simulink library "breakers_1ph_3ph"  (R2013a)
settings: Solver=ode45  StartTime=0.0  StopTime=10.0  RelTol=1e-3
undefined symbols (not defined in the file): DiscIntNeverNeededParam, IOC, sim_Freq_Hz, TOC, TOC_T, Ts
libraries: simulink x8, powerlib_extras x7, breakers_1ph_3ph x4, simulink_extras x4, powerlib x4, dspsigops x3
settings Model: Creator=re25624  LastModifiedBy=ed12083

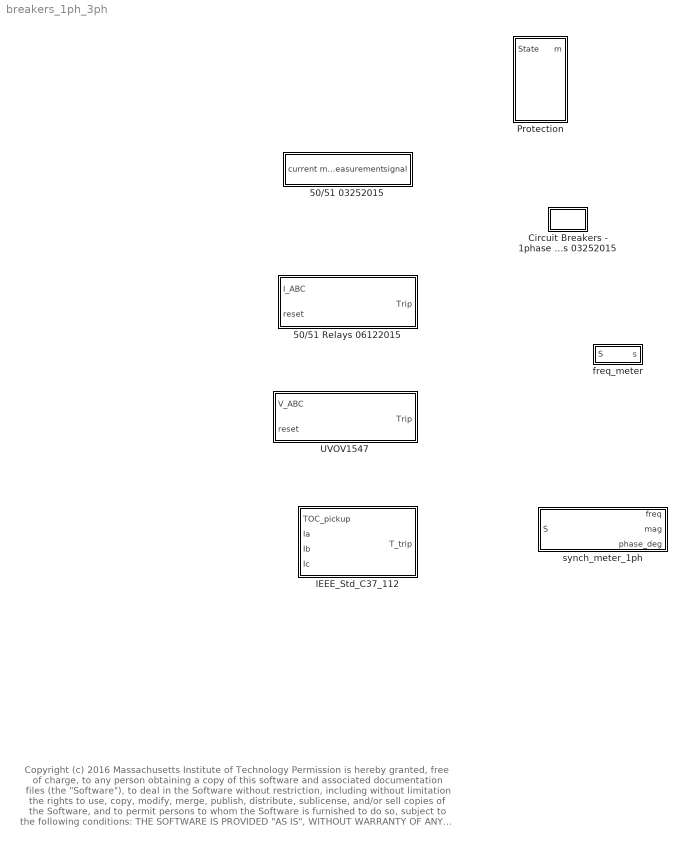
== system breakers_1ph_3ph ==
  note: Copyright (c) 2016 Massachusetts Institute of Technology
      | Permission is hereby granted, free of charge, to any person obtaining a copy of this software and associated documentation files (the "Software"), to deal
      | in the Software without restriction, including without limitation the rights to use, copy, modify, merge, publish, distribute, sublicense, and/or sell copies of the
      | Software, and to permit persons to whom the Software is furnished to do so, subject to the following conditions:
      |
      | THE SOFTWARE IS PROVIDED "AS IS", WITHOUT WARRANTY OF ANY KIND, EXPRESS OR IMPLIED, INCLUDING BUT NOT LIMITED TO THE
      | WARRANTIES OF MERCHANTABILITY, FITNESS FOR A PARTICULAR PURPOSE AND NONINFRINGEMENT. IN NO EVENT SHALL THE AUTHORS
      | OR COPYRIGHT HOLDERS BE LIABLE FOR ANY CLAIM, DAMAGES OR OTHER LIABILITY, WHETHER IN AN ACTION OF CONTRACT, TORT OR
      | OTHERWISE, ARISING FROM, OUT OF OR IN CONNECTION WITH THE SOFTWARE OR THE USE OR OTHER DEALINGS IN THE SOFTWARE
  50/51 03252015 : Subsystem  mask{IOC=IOC, TOC=TOC, TOC_T=TOC_T, Ts=Ts, sim_Freq_Hz=sim_Freq_Hz}
      mask prompts: IOC "IOC [A]"; TOC "TOC [A]"; TOC_T "TOC Delay [Sec]"; Ts "Sampling Time"; sim_Freq_Hz "Frequency [Hz]"
      mask help: This is a very simple model of instantaneous overcurrent and the inverse time overcurrent relays (50/51). It is not suitable for instantaneous earth current relaying. The model neglects the influence CTs since only the logics of the relay are required or the current effort. The input parameters to the model are: measured line current, sampling time (Ts) and simulation frequency (sim_Freq_Hz)
  50/51 Relays 06122015 : Subsystem  mask(50/51 Relays){TOC=150, IOC=900, Ts=Ts}
      mask prompts: TOC "TOC [A]"; IOC "IOC [A]"; Ts "Sampling Time [Secs]"
      mask help:
      | This is a model of instantaneous overcurrent and the inverse time overcurrent relays (50/51).
      | It is not suitable for instantaneous earth current relaying.
      | The model neglects the influence CTs since only the logics of the relay are required or the current effort.
      | The input parameters to the model are: measured line current, and sampling time (Ts)
  Circuit Breakers - 1phase with 50/51 relays 03252015 : Subsystem  mask{IOC=3000, TOC=600, TOC_T=0.1, MECH_T=0.05, open_command=1E15, close_command=1E15, sim_Freq_Hz=60, Ts=50e-6}
      mask prompts: IOC "IOC setting [A]"; TOC "TOC setting [A]"; TOC_T "TOC time dealy [Sec]"; MECH_T "Mechanical time delay [Sec]"; open_command "Manual open time [Sec]"; close_command "Manual close time [Sec]"; sim_Freq_Hz "Frequency [Hz]"; Ts "Sampling Time"
  IEEE_Std_C37_112 : Subsystem
  Protection : Subsystem  mask(Protection and Metering){IOC=7200, TOC=1920, Ts=50E-6}
      mask prompts: IOC "IOC setting [A]"; TOC "TOC setting [A]"; Ts "Sampling Time"
      mask help:
      | This block simulates the behavior of selected relay functions as well as metering equipment.
      | The block is intended to communicate with a microgrid controller providing it measurements, and switching controls.
      |
      | Supported relay functions (as of 06-15-2015):
      | 50/51: instantaneous and time-inverse overcurrent protection (moderate curve)
      mask Help:
      | This block simulates the behavior of selected relay functions as well as metering equipment (60 Hz - only).
      | The block is intended to communicate with a microgrid controller providing it measurements, and switching controls.
      | 
      | Supported relay functions (as of 06-15-2015):
      | 50/51: instantaneous and time-inverse overcurrent protection (moderate curve)
      | 
      | The input parameters are:
      | 0) Ts:  Sampling time [Seconds]
      | 1) State: 0 for relay logic mode, 1 to close the controlled breaker/switch,
      | and 2 to open the controlled breaker/switch
      | 2) TOC: Time-inverse overcurrent setting [Amperes]
      | 3) IOC: Instantaneous overcurrent setting [Amperes]
      | 
      | Metered parameters are:
      | 0) Status (0-closed, 1-open)
      | 1) Instantaneous voltage (abc)
      | 2) Instantaneous current (abc)
  UVOV1547 : Subsystem  mask(IEEE Std. 1457 UVOV Protection){VRMSLL=13800, Ts=Ts}
      mask prompts: VRMSLL "Nominal Voltage [VRMSLL]"; Ts "Sampling Time, [Secs]"
      mask help:
      | This is a model of the IEEE Std. 1457 undervoltage and overvoltage protection check.
      | The model neglects the influence PTs since only the logics of the relay are required or the current effort.
      | The input parameters to the model are: measured voltage RMSLL, and sampling time (Ts)
  freq_meter : Subsystem  mask(Frequency Meter){Ts=Ts}
      mask prompts: Ts "Time Step, Ts [Sec]"
      mask help:
      | This block measures the frequency of and input signal (voltage, current, etc) at the rising edge of zero-crossing. There more advanced and efficient methods to meter frequency (i.e. DFT). However, most of the relays in the power system operate on the principle of zero crossing detection.
      |
      | ** The error in measurement is relative to the specified time step. It is recommended Ts <= 80E-6 s.
  synch_meter_1ph : Subsystem  mask(Synchronizer meter){Ts=Ts}
      mask prompts: Ts "Time Step, Ts [sec]"
      mask help:
      | This block measures frequency, magnitude and phase of an input signal. Requires one cycle to initialize.
      | **** The error in measurement of the internal components is relative to the specified time step. It is recommended Ts <= 80E-6 s.

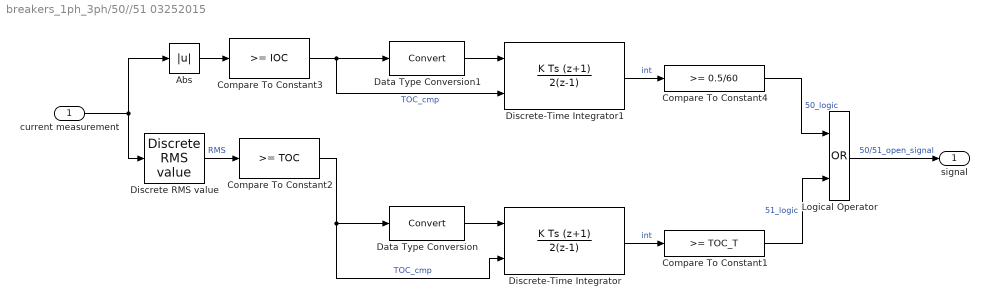
== system breakers_1ph_3ph/50//51 03252015 ==
  current measurement : Inport
  Abs : Abs
  Compare To Constant1 : simulink/Logic and Bit Operations/Compare To Constant  relop=>=  const=TOC_T  OutDataTypeStr=boolean
  Compare To Constant2 : simulink/Logic and Bit Operations/Compare To Constant  relop=>=  const=TOC  OutDataTypeStr=boolean
  Compare To Constant3 : simulink/Logic and Bit Operations/Compare To Constant  relop=>=  const=IOC  OutDataTypeStr=boolean
  Compare To Constant4 : simulink/Logic and Bit Operations/Compare To Constant  relop=>=  const=0.5/60  OutDataTypeStr=boolean
  Data Type Conversion : DataTypeConversion
  Data Type Conversion1 : DataTypeConversion
  Discrete RMS value : powerlib_extras/Discrete Measurements/Discrete  RMS value  Freq=60  Mag_Init=0  Ts=Ts
  Discrete-Time Integrator : DiscreteIntegrator  IntegratorMethod=Integration: Trapezoidal  ExternalReset=falling  InitialConditionMode=State only (most efficient)  SampleTime=-1  ICPrevOutput=DiscIntNeverNeededParam  ICPrevScaledInput=DiscIntNeverNeededParam
  Discrete-Time Integrator1 : DiscreteIntegrator  IntegratorMethod=Integration: Trapezoidal  ExternalReset=falling  InitialConditionMode=State only (most efficient)  SampleTime=-1  ICPrevOutput=DiscIntNeverNeededParam  ICPrevScaledInput=DiscIntNeverNeededParam
  Logical Operator : Logic  Operator=OR  AllPortsSameDT=off  OutDataTypeStr=boolean
  signal : Outport
  wires:
  Logical Operator/1 -> signal/1  "50/51_open_signal"
  Compare To Constant1/1 -> Logical Operator/2  "51_logic"
  Abs/1 -> Compare To Constant3/1
  Discrete RMS value/1 -> Compare To Constant2/1  "RMS"
  Data Type Conversion/1 -> Discrete-Time Integrator/1
  Discrete-Time Integrator/1 -> Compare To Constant1/1  "int"
  current measurement/1 -> Abs/1, Discrete RMS value/1
  Compare To Constant2/1 -> Discrete-Time Integrator/2, Data Type Conversion/1  "TOC_cmp"
  Data Type Conversion1/1 -> Discrete-Time Integrator1/1
  Discrete-Time Integrator1/1 -> Compare To Constant4/1  "int"
  Compare To Constant3/1 -> Discrete-Time Integrator1/2, Data Type Conversion1/1  "TOC_cmp"
  Compare To Constant4/1 -> Logical Operator/1  "50_logic"

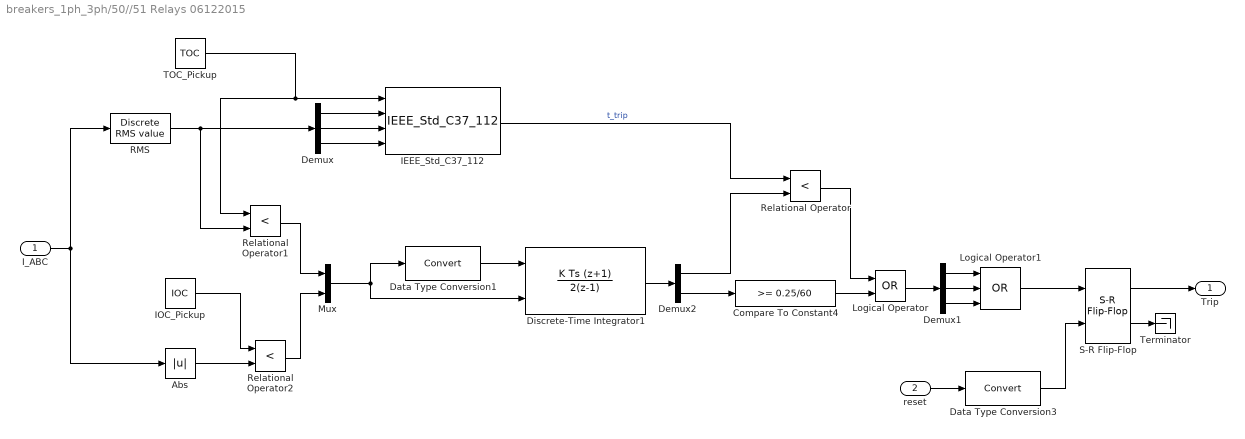
== system breakers_1ph_3ph/50//51 Relays 06122015 ==
  I_ABC : Inport
  reset : Inport  Port=2
  Abs : Abs
  Compare To Constant4 : simulink/Logic and Bit Operations/Compare To Constant  relop=>=  const=0.25/60  OutDataTypeStr=boolean
  Data Type Conversion1 : DataTypeConversion
  Data Type Conversion3 : DataTypeConversion
  Demux : Demux  Outputs=3
  Demux1 : Demux  Outputs=3
  Demux2 : Demux  Outputs=2
  Discrete-Time Integrator1 : DiscreteIntegrator  IntegratorMethod=Integration: Trapezoidal  ExternalReset=falling  InitialConditionMode=State only (most efficient)  SampleTime=-1  ICPrevOutput=DiscIntNeverNeededParam  ICPrevScaledInput=DiscIntNeverNeededParam
  IEEE_Std_C37_112 : breakers_1ph_3ph/IEEE_Std_C37_112
  IOC_Pickup : Constant  Value=IOC
  Logical Operator : Logic  Operator=OR  AllPortsSameDT=off  OutDataTypeStr=boolean
  Logical Operator1 : Logic  Operator=OR  Inputs=3  AllPortsSameDT=off  OutDataTypeStr=boolean
  Mux : Mux  Inputs=2
  RMS : powerlib_extras/Discrete Measurements/Discrete  RMS value  Freq=60  Mag_Init=0  Ts=Ts
  Relational Operator : RelationalOperator  Operator=<  OutDataTypeStr=boolean
  Relational Operator1 : RelationalOperator  Operator=<  OutDataTypeStr=boolean
  Relational Operator2 : RelationalOperator  Operator=<  OutDataTypeStr=boolean
  S-R Flip-Flop : simulink_extras/Flip Flops/S-R Flip-Flop  initial_condition=0
  TOC_Pickup : Constant  Value=TOC
  Terminator : Terminator
  Trip : Outport
  wires:
  Demux2/2 -> Compare To Constant4/1
  Demux2/1 -> Relational Operator/2
  Discrete-Time Integrator1/1 -> Demux2/1
  Mux/1 -> Discrete-Time Integrator1/2, Data Type Conversion1/1
  Relational Operator2/1 -> Mux/2
  Relational Operator1/1 -> Mux/1
  Data Type Conversion3/1 -> S-R Flip-Flop/2
  reset/1 -> Data Type Conversion3/1
  Logical Operator1/1 -> S-R Flip-Flop/1
  Demux1/3 -> Logical Operator1/3
  Demux1/2 -> Logical Operator1/2
  Demux1/1 -> Logical Operator1/1
  Logical Operator/1 -> Demux1/1
  S-R Flip-Flop/2 -> Terminator/1
  S-R Flip-Flop/1 -> Trip/1
  I_ABC/1 -> RMS/1, Abs/1
  TOC_Pickup/1 -> Relational Operator1/1, IEEE_Std_C37_112/1
  Demux/3 -> IEEE_Std_C37_112/4
  Demux/2 -> IEEE_Std_C37_112/3
  Demux/1 -> IEEE_Std_C37_112/2
  RMS/1 -> Relational Operator1/2, Demux/1
  IOC_Pickup/1 -> Relational Operator2/1
  Relational Operator/1 -> Logical Operator/1
  Compare To Constant4/1 -> Logical Operator/2
  Abs/1 -> Relational Operator2/2
  IEEE_Std_C37_112/1 -> Relational Operator/1  "t_trip"
  Data Type Conversion1/1 -> Discrete-Time Integrator1/1

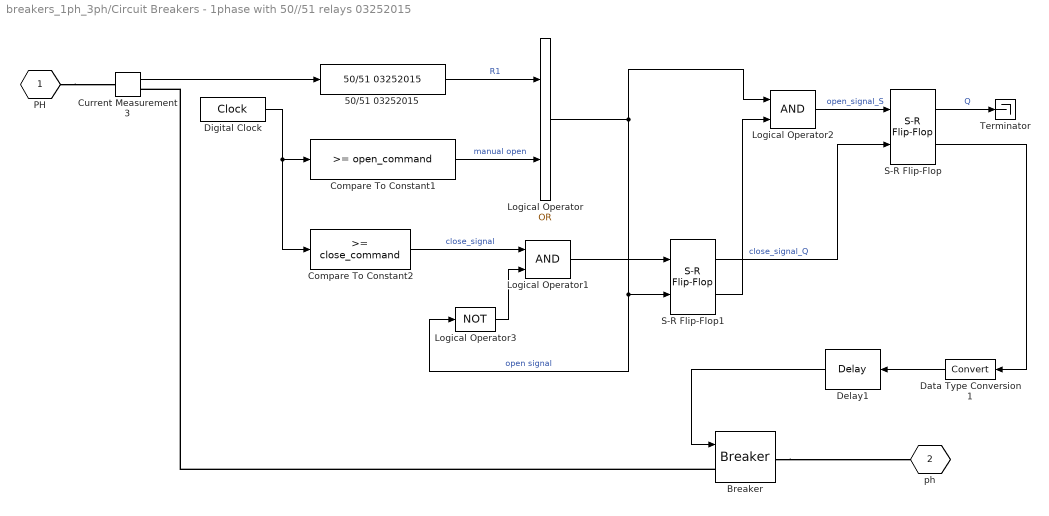
== system breakers_1ph_3ph/Circuit Breakers - 1phase with 50//51 relays 03252015 ==
  50/51 03252015 : breakers_1ph_3ph/50//51 03252015  IOC=IOC  TOC=TOC  TOC_T=TOC_T  Ts=Ts  sim_Freq_Hz=sim_Freq_Hz
  Breaker : powerlib/Elements/Breaker  BreakerResistance=1e-3  InitialState=1  SnubberResistance=1e6  SnubberCapacitance=inf  SwitchingTimes="[1/60  5/60]"  External=on  Measurements=None  MoreParameters=on  NoBreakLoop=off
  Compare To Constant1 : simulink/Logic and Bit Operations/Compare To Constant  relop=>=  const=open_command  OutDataTypeStr=boolean
  Compare To Constant2 : simulink/Logic and Bit Operations/Compare To Constant  relop=>=  const=close_command  OutDataTypeStr=boolean
  Current Measurement3 : powerlib/Measurements/Current Measurement  PhasorSimulation=off  OutputType=Complex  PSBequivalent=0
  Data Type Conversion1 : DataTypeConversion
  Delay1 : dspsigops/Delay  dly_unit=Samples  delay=lower(MECH_T/Ts)  ic_detail=off  dif_ic_for_ch=off  dif_ic_for_dly=off  ic=1  reset_popup=None
  Digital Clock : DigitalClock  SampleTime=Ts
  Logical Operator : Logic  Operator=OR  AllPortsSameDT=off  OutDataTypeStr=boolean
  Logical Operator1 : Logic  AllPortsSameDT=off  OutDataTypeStr=boolean
  Logical Operator2 : Logic  AllPortsSameDT=off  OutDataTypeStr=boolean
  Logical Operator3 : Logic  Operator=NOT  AllPortsSameDT=off  OutDataTypeStr=boolean
  S-R Flip-Flop : simulink_extras/Flip Flops/S-R Flip-Flop  initial_condition=0
  S-R Flip-Flop1 : simulink_extras/Flip Flops/S-R Flip-Flop  initial_condition=0
  Terminator : Terminator
  PH : PMIOPort  Tag=PMCPort  Port=1  Side=Left
  ph : PMIOPort  Tag=PMCPort  Port=2  Side=Right
  wires:
  Delay1/1 -> Breaker/1
  Logical Operator1/1 -> S-R Flip-Flop1/1
  Compare To Constant2/1 -> Logical Operator1/1  "close_signal"
  Logical Operator/1 -> S-R Flip-Flop1/2, Logical Operator3/1, Logical Operator2/1  "open signal"
  S-R Flip-Flop1/1 -> S-R Flip-Flop/2  "close_signal_Q"
  S-R Flip-Flop/2 -> Data Type Conversion1/1
  S-R Flip-Flop1/2 -> Logical Operator2/2
  Compare To Constant1/1 -> Logical Operator/2  "manual open"
  Logical Operator3/1 -> Logical Operator1/2
  Digital Clock/1 -> Compare To Constant1/1, Compare To Constant2/1
  50/51 03252015/1 -> Logical Operator/1  "R1"
  S-R Flip-Flop/1 -> Terminator/1  "Q"
  Current Measurement3/1 -> 50/51 03252015/1
  Logical Operator2/1 -> S-R Flip-Flop/1  "open_signal_S"
  Data Type Conversion1/1 -> Delay1/1
  connections:
  Breaker/RConn1 -- ph/RConn1
  PH/RConn1 -- Current Measurement3/LConn1
  Breaker/LConn1 -- Current Measurement3/RConn1

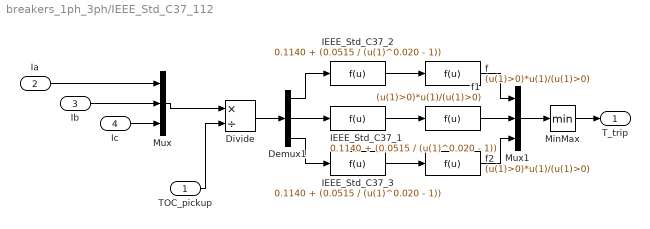
== system breakers_1ph_3ph/IEEE_Std_C37_112 ==
  TOC_pickup : Inport
  Ia : Inport  Port=2
  Ib : Inport  Port=3
  Ic : Inport  Port=4
  Demux1 : Demux  Outputs=3
  Divide : Product  Inputs=*/
  IEEE_Std_C37_1 : Fcn  Expr=0.1140 + (0.0515 / (u(1)^0.020 - 1))
  IEEE_Std_C37_2 : Fcn  Expr=0.1140 + (0.0515 / (u(1)^0.020 - 1))
  IEEE_Std_C37_3 : Fcn  Expr=0.1140 + (0.0515 / (u(1)^0.020 - 1))
  MinMax : MinMax
  Mux : Mux  Inputs=3
  Mux1 : Mux  Inputs=3
  f : Fcn  Expr=(u(1)>0)*u(1)/(u(1)>0)
  f1 : Fcn  Expr=(u(1)>0)*u(1)/(u(1)>0)
  f2 : Fcn  Expr=(u(1)>0)*u(1)/(u(1)>0)
  T_trip : Outport
  wires:
  Ic/1 -> Mux/3
  TOC_pickup/1 -> Divide/2
  MinMax/1 -> T_trip/1
  Ib/1 -> Mux/2
  Ia/1 -> Mux/1
  f2/1 -> Mux1/3
  f1/1 -> Mux1/2
  f/1 -> Mux1/1
  Mux/1 -> Divide/1
  Mux1/1 -> MinMax/1
  IEEE_Std_C37_3/1 -> f2/1
  IEEE_Std_C37_1/1 -> f1/1
  IEEE_Std_C37_2/1 -> f/1
  Divide/1 -> Demux1/1
  Demux1/3 -> IEEE_Std_C37_3/1
  Demux1/2 -> IEEE_Std_C37_1/1
  Demux1/1 -> IEEE_Std_C37_2/1

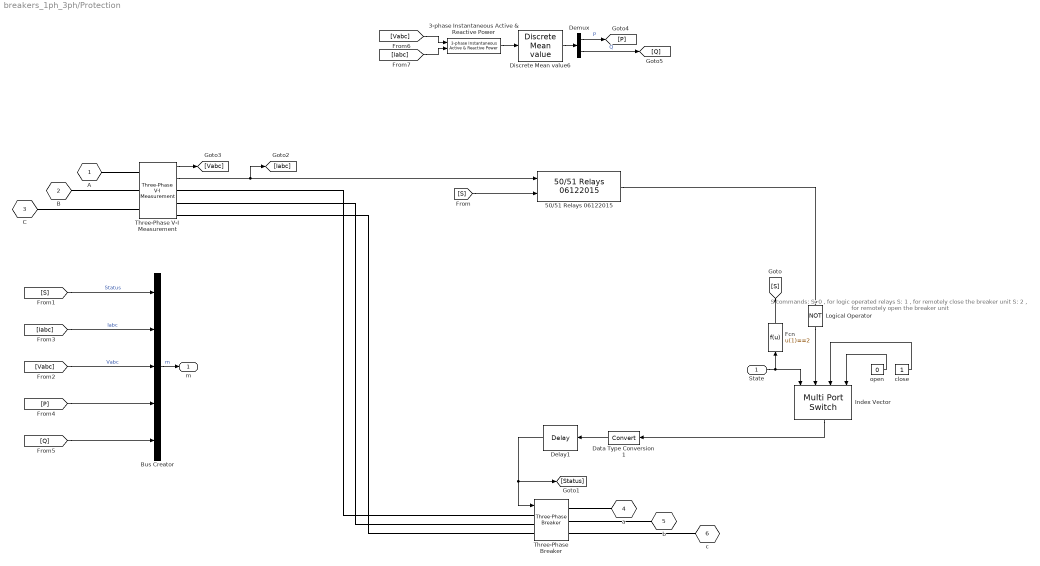
== system breakers_1ph_3ph/Protection ==
  note: S commands:
      | S: 0 , for logic operated relays
      | S: 1 ,  for remotely close the breaker unit
      | S: 2 , for remotely open the breaker unit
  State : Inport
  3-phase Instantaneous Active & Reactive Power : powerlib_extras/Measurements/3-phase  Instantaneous  Active & Reactive Power
  50/51 Relays 06122015 : breakers_1ph_3ph/50//51 Relays 06122015  TOC=TOC  IOC=IOC  Ts=Ts
  Bus Creator : BusCreator  Inputs=5
  Data Type Conversion1 : DataTypeConversion
  Delay1 : dspsigops/Delay  dly_unit=Samples  delay=lower((3/60)/Ts)  ic_detail=off  dif_ic_for_ch=off  dif_ic_for_dly=off  ic=1  reset_popup=None
  Demux : Demux  Outputs=2
  Discrete Mean value6 : powerlib_extras/Discrete Measurements/Discrete  Mean value  Freq=60  Vinit=0  Ts=Ts
  Fcn : Fcn  Expr=u(1)==2
  Index Vector : MultiPortSwitch  DataPortOrder=Zero-based contiguous  DataPortIndices={2,1,0}  zeroidx=on
  Logical Operator : Logic  Operator=NOT  AllPortsSameDT=off  OutDataTypeStr=boolean
  Three-Phase V-I Measurement : powerlib/Measurements/Three-Phase V-I Measurement  VoltageMeasurement=phase-to-ground  SetLabelV=off  LabelV=Vabc  Vpu=off  VpuLL=off  CurrentMeasurement=yes  SetLabelI=off  LabelI=Iabc  Ipu=off  Pbase=100e6  Vbase=500e3  OutputType=Complex  PhasorSimulation=off  PSBequivalent=0
  Three-Phase Breaker : powerlib/Elements/Three-Phase Breaker  InitialState=closed  SwitchA=on  SwitchB=on  SwitchC=on  SwitchTimes="[1/60  5/60]"  External=on  BreakerResistance=1e-3  SnubberResistance=1e6  SnubberCapacitance=1e-12  Measurements=None
  close : Constant
  open : Constant  Value=0
  A : PMIOPort  Tag=PMCPort  Port=1  Side=Left
  B : PMIOPort  Tag=PMCPort  Port=2  Side=Left
  C : PMIOPort  Tag=PMCPort  Port=3  Side=Left
  a : PMIOPort  Tag=PMCPort  Port=4  Side=Right
  b : PMIOPort  Tag=PMCPort  Port=5  Side=Right
  c : PMIOPort  Tag=PMCPort  Port=6  Side=Right
  m : Outport
  wires:
  Data Type Conversion1/1 -> Delay1/1
  Index Vector/1 -> Data Type Conversion1/1
  State/1 -> Index Vector/1, Fcn/1
  close/1 -> Index Vector/3
  open/1 -> Index Vector/4
  Three-Phase V-I Measurement/2 -> 50/51 Relays 06122015/1, [Iabc]
  Three-Phase V-I Measurement/1 -> [Vabc]
  Delay1/1 -> Three-Phase Breaker/1, [Status]
  [S] -> 50/51 Relays 06122015/2
  [S] -> Bus Creator/1  "Status"
  Bus Creator/1 -> m/1  "m"
  Fcn/1 -> [S]
  Logical Operator/1 -> Index Vector/2
  50/51 Relays 06122015/1 -> Logical Operator/1
  Discrete Mean value6/1 -> Demux/1
  3-phase Instantaneous Active & Reactive Power/1 -> Discrete Mean value6/1
  Demux/2 -> [Q]  "Q"
  Demux/1 -> [P]  "P"
  [Iabc] -> Bus Creator/2  "Iabc"
  [Vabc] -> Bus Creator/3  "Vabc"
  [Iabc] -> 3-phase Instantaneous Active & Reactive Power/2
  [Vabc] -> 3-phase Instantaneous Active & Reactive Power/1
  [P] -> Bus Creator/4
  [Q] -> Bus Creator/5
  connections:
  B/RConn1 -- Three-Phase V-I Measurement/LConn2
  C/RConn1 -- Three-Phase V-I Measurement/LConn3
  a/RConn1 -- Three-Phase Breaker/RConn1
  Three-Phase V-I Measurement/LConn1 -- A/RConn1
  Three-Phase Breaker/RConn3 -- c/RConn1
  Three-Phase Breaker/RConn2 -- b/RConn1
  Three-Phase Breaker/LConn3 -- Three-Phase V-I Measurement/RConn3
  Three-Phase Breaker/LConn2 -- Three-Phase V-I Measurement/RConn2
  Three-Phase Breaker/LConn1 -- Three-Phase V-I Measurement/RConn1

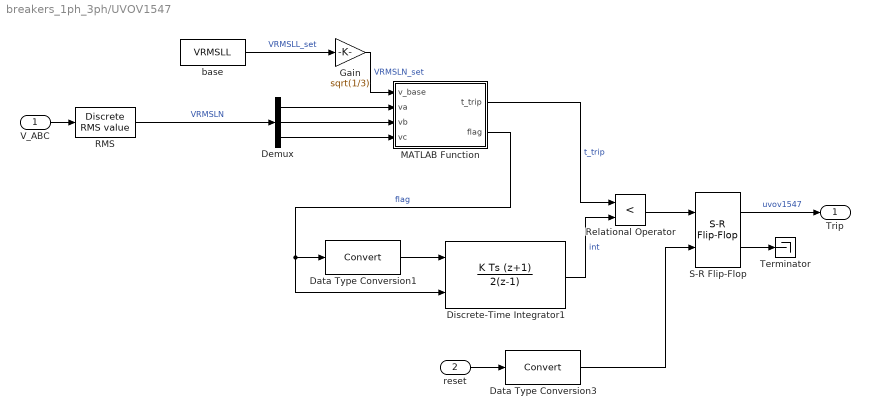
== system breakers_1ph_3ph/UVOV1547 ==
  V_ABC : Inport
  reset : Inport  Port=2
  Data Type Conversion1 : DataTypeConversion
  Data Type Conversion3 : DataTypeConversion
  Demux : Demux  Outputs=3
  Discrete-Time Integrator1 : DiscreteIntegrator  IntegratorMethod=Integration: Trapezoidal  ExternalReset=falling  InitialConditionMode=State only (most efficient)  SampleTime=-1  ICPrevOutput=DiscIntNeverNeededParam  ICPrevScaledInput=DiscIntNeverNeededParam
  Gain : Gain  Gain=sqrt(1/3)
  MATLAB Function : MATLAB Function  TreatAsAtomicUnit=on
  RMS : powerlib_extras/Discrete Measurements/Discrete  RMS value  Freq=60  Mag_Init=VRMSLL*sqrt(1/3)  Ts=Ts
  Relational Operator : RelationalOperator  Operator=<  OutDataTypeStr=boolean
  S-R Flip-Flop : simulink_extras/Flip Flops/S-R Flip-Flop  initial_condition=0
  Terminator : Terminator
  base : Constant  Value=VRMSLL
  Trip : Outport
  wires:
  V_ABC/1 -> RMS/1
  Relational Operator/1 -> S-R Flip-Flop/1
  MATLAB Function/2(flag) -> Discrete-Time Integrator1/2, Data Type Conversion1/1  "flag"
  Gain/1 -> MATLAB Function/1(v_base)  "VRMSLN_set"
  Discrete-Time Integrator1/1 -> Relational Operator/2  "int"
  Data Type Conversion3/1 -> S-R Flip-Flop/2
  reset/1 -> Data Type Conversion3/1
  S-R Flip-Flop/2 -> Terminator/1
  S-R Flip-Flop/1 -> Trip/1  "uvov1547"
  base/1 -> Gain/1  "VRMSLL_set"
  Demux/3 -> MATLAB Function/4(vc)
  Demux/2 -> MATLAB Function/3(vb)
  Demux/1 -> MATLAB Function/2(va)
  RMS/1 -> Demux/1  "VRMSLN"
  MATLAB Function/1(t_trip) -> Relational Operator/1  "t_trip"
  Data Type Conversion1/1 -> Discrete-Time Integrator1/1

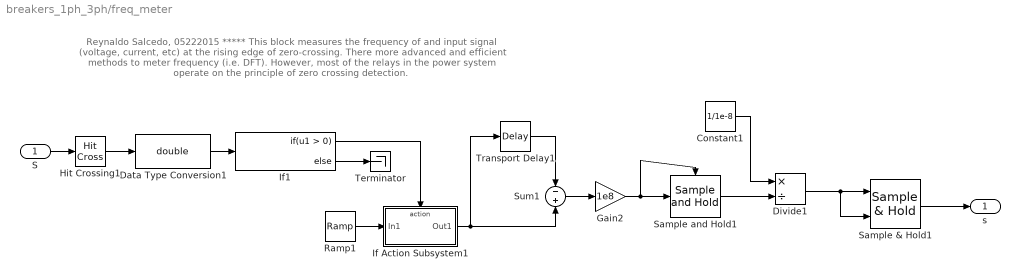
== system breakers_1ph_3ph/freq_meter ==
  note: Reynaldo Salcedo, 05222015
      | ***** This block measures the frequency of and input signal (voltage, current, etc) at the rising edge of zero-crossing.
      | There more advanced and efficient methods to meter frequency (i.e. DFT).
      | However, most of the relays in the power system operate on the principle of zero crossing detection.
  S : Inport
  Constant1 : Constant  Value=1/1e-8
  Data Type Conversion1 : DataTypeConversion  OutDataTypeStr=double
  Divide1 : Product  Inputs=*/
  Gain2 : Gain  Gain=1e8
  Hit Crossing1 : HitCross  HitCrossingDirection=rising
  If Action Subsystem1 : Subsystem  TreatAsAtomicUnit=on
  If1 : If
  Ramp1 : simulink/Sources/Ramp  slope=1  start=0  X0=60
  Sample and Hold1 : dspsigops/Sample and Hold  trig=Rising edge  initCond=0  latchinput=off
  Sample & Hold1 : powerlib_extras/Control  Blocks/Sample & Hold  ic=0
  Sum1 : Sum  Inputs=-+
  Terminator : Terminator
  Transport Delay1 : TransportDelay  DelayTime=Ts
  s : Outport
  wires:
  Sample and Hold1/1 -> Divide1/2
  Divide1/1 -> Sample & Hold1/2, Sample & Hold1/1
  If1/2 -> Terminator/1
  If1/1 -> If Action Subsystem1/Action
  Sample & Hold1/1 -> s/1
  Constant1/1 -> Divide1/1
  Gain2/1 -> Sample and Hold1/Trigger, Sample and Hold1/1
  Sum1/1 -> Gain2/1
  Transport Delay1/1 -> Sum1/1
  If Action Subsystem1/1(Out1) -> Sum1/2, Transport Delay1/1
  Ramp1/1 -> If Action Subsystem1/1(In1)
  Hit Crossing1/1 -> Data Type Conversion1/1
  Data Type Conversion1/1 -> If1/1
  S/1 -> Hit Crossing1/1

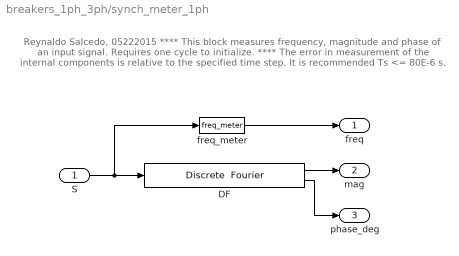
== system breakers_1ph_3ph/synch_meter_1ph ==
  note: Reynaldo Salcedo, 05222015
      | **** This block measures frequency, magnitude and phase of an input signal.
      | Requires one cycle to initialize.
      | **** The error in measurement of the internal components is relative to the specified time step. It is recommended Ts <= 80E-6 s.
  S : Inport
  DF : powerlib_extras/Discrete Measurements/Discrete  Fourier  Freq=60  n=1  Par_Init=[0 0]  Ts=Ts
  freq_meter : breakers_1ph_3ph/freq_meter  Ts=Ts
  freq : Outport
  mag : Outport  Port=2
  phase_deg : Outport  Port=3
  wires:
  S/1 -> DF/1, freq_meter/1
  freq_meter/1 -> freq/1
  DF/2 -> phase_deg/1
  DF/1 -> mag/1

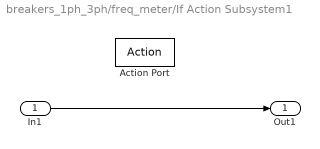
== system breakers_1ph_3ph/freq_meter/If Action Subsystem1 ==
  In1 : Inport
  Action Port : ActionPort
  Out1 : Outport
  wires:
  In1/1 -> Out1/1

== matlab function breakers_1ph_3ph/UVOV1547/MATLAB Function ==
  data: v_base input; va input; t_trip output; vb input; vc input; flag output
function [t_trip, flag] = uvov1547(v_base,va,vb,vc)
%#codegen

v_pu = [va, vb, vc] ./ v_base;
mech_delay = 3/60;
t = 1E6;
flag = 0;

% IEEE Std 1547a-2014 (Amendment to IEEE Std 1547-2003)
% Table 1-Interconnection system default response to abnormal voltages

if max(v_pu < 0.45)
    t=0.16;
    flag=1;
elseif max(v_pu >= 0.45) && max(v_pu < 0.60)
    t=1;
    flag=1;
elseif max(v_pu >= 0.60) && max(v_pu < 0.88)
    t=2;
    flag=1;
elseif max(v_pu >= 1.10) && max(v_pu < 1.20)
    t=1;
    flag=1;
elseif max(v_pu >= 1.20)
    t=0.16;
    flag=1;
end

t_trip = abs(t - mech_delay);
